simulink model "chris_4R_all_primitives"  (R2024b)
settings: Solver=FixedStepDiscrete  StartTime=0.0  StopTime=60  FixedStep=0.1  MaxStep=0.1  RelTol=1e-3
libraries: neural x220, simulink x1, realtime_pacer_lib x1
(part 8 of 9)

== system chris_4R_all_primitives/RGB to HSV to vel - all robots4/Hue Neural Network/Layer 3/Delays 1 ==
  "p{3}" : Inport  PortDimensions=7
      mask Display: e = 0.06;c1 = [120 230 180]/255;c2 = ([120 230 180]+0)/(256+128);c3 = ([120 230 180]+128)/(256+128);patch([0 1 1 0],[0 0 1 1],c1);patch([0 1 1 1-e 1-e 0+e],[0 0 1 1-e 0+e 0+e],c2);patch([0 0 1 1-e 0+e 0+e],[0 1 1 1-e 1-e 0+e],c3);plot([0 1 1 0 0],[0 0 1 1 0]);
  mux : Mux  Inputs=1
      mask Display: e = 0.06;c1 = [120 150 230]/255;c2 = ([120 150 230]+0)/383;c3 = ([120 150 230]+128)/383;patch([0 1 1 0],[0 0 1 1],c1);patch([0 1 1 1-e 1-e 0+e],[0 0 1 1-e 0+e 0+e],c2);patch([0 0 1 1-e 0+e 0+e],[0 1 1 1-e 1-e 0+e],c3);plot([0 1 1 0 0],[0 0 1 1 0]);disp('Mux')
  "pd{3,2}" : Outport
      mask Display: e = 0.06;c1 = [120 230 180]/255;c2 = ([120 230 180]+0)/(256+128);c3 = ([120 230 180]+128)/(256+128);patch([0 1 1 0],[0 0 1 1],c1);patch([0 1 1 1-e 1-e 0+e],[0 0 1 1-e 0+e 0+e],c2);patch([0 0 1 1-e 0+e 0+e],[0 1 1 1-e 1-e 0+e],c3);plot([0 1 1 0 0],[0 0 1 1 0]);
  wires:
  "p{3}"/1 -> mux/1
  mux/1 -> "pd{3,2}"/1

== system chris_4R_all_primitives/RGB to HSV to vel - all robots4/Hue Neural Network/Layer 3/LW{3,2} ==
  "ad{3,2}" : Inport  PortDimensions=7
      mask Display: e = 0.06;c1 = [120 230 180]/255;c2 = ([120 230 180]+0)/(256+128);c3 = ([120 230 180]+128)/(256+128);patch([0 1 1 0],[0 0 1 1],c1);patch([0 1 1 1-e 1-e 0+e],[0 0 1 1-e 0+e 0+e],c2);patch([0 0 1 1-e 0+e 0+e],[0 1 1 1-e 1-e 0+e],c3);plot([0 1 1 0 0],[0 0 1 1 0]);
  "IW{3,2}(1,:)'" : Constant  Value=[0.2692392715730551611130749734002165496349334716796875;0.176447254974731071452964670243090949952602386474609375;-0.2006583795199970710054770961505710147321224212646484375;0.116348530779392056455634474332327954471111297607421875;0.052531073636257800962834352276331628672778606414794921875;0.02289851615612122082143997658931766636669635772705078125;0.55928841319732980341683514780015684664249420166015625]
      mask Display: e = 0.06;c1 = [120 150 230]/255;c2 = ([120 150 230]+0)/383;c3 = ([120 150 230]+128)/383;patch([0 1 1 0],[0 0 1 1],c1);patch([0 1 1 1-e 1-e 0+e],[0 0 1 1-e 0+e 0+e],c2);patch([0 0 1 1-e 0+e 0+e],[0 1 1 1-e 1-e 0+e],c3);plot([0 1 1 0 0],[0 0 1 1 0]);disp('weights');
  "IW{3,2}(2,:)'" : Constant  Value=[0.2331519658198511202318314872172777540981769561767578125;-0.06009291383108665562939876281234319321811199188232421875;0.440376448501252071299205681498278863728046417236328125;-0.0075677260182224516393834079508451395668089389801025390625;0.3030442642604487257784739995258860290050506591796875;-0.2185483415876194601690230001622694544494152069091796875;0.11610241287844720592392633307099458761513233184814453125]
      mask Display: e = 0.06;c1 = [120 150 230]/255;c2 = ([120 150 230]+0)/383;c3 = ([120 150 230]+128)/383;patch([0 1 1 0],[0 0 1 1],c1);patch([0 1 1 1-e 1-e 0+e],[0 0 1 1-e 0+e 0+e],c2);patch([0 0 1 1-e 0+e 0+e],[0 1 1 1-e 1-e 0+e],c3);plot([0 1 1 0 0],[0 0 1 1 0]);disp('weights');
  Mux : Mux  Inputs=2
      mask Display: e = 0.06;c1 = [120 150 230]/255;c2 = ([120 150 230]+0)/383;c3 = ([120 150 230]+128)/383;patch([0 1 1 0],[0 0 1 1],c1);patch([0 1 1 1-e 1-e 0+e],[0 0 1 1-e 0+e 0+e],c2);patch([0 0 1 1-e 0+e 0+e],[0 1 1 1-e 1-e 0+e],c3);plot([0 1 1 0 0],[0 0 1 1 0]);disp('Mux');
  dotprod1 : neural/Weight Functions/dotprod
  dotprod2 : neural/Weight Functions/dotprod
  "lz{3,2}" : Outport
      mask Display: e = 0.06;c1 = [120 230 180]/255;c2 = ([120 230 180]+0)/(256+128);c3 = ([120 230 180]+128)/(256+128);patch([0 1 1 0],[0 0 1 1],c1);patch([0 1 1 1-e 1-e 0+e],[0 0 1 1-e 0+e 0+e],c2);patch([0 0 1 1-e 0+e 0+e],[0 1 1 1-e 1-e 0+e],c3);plot([0 1 1 0 0],[0 0 1 1 0]);
  wires:
  "IW{3,2}(1,:)'"/1 -> dotprod1/1
  "ad{3,2}"/1 -> dotprod1/2, dotprod2/2
  dotprod1/1 -> Mux/1
  "IW{3,2}(2,:)'"/1 -> dotprod2/1
  dotprod2/1 -> Mux/2
  Mux/1 -> "lz{3,2}"/1

== system chris_4R_all_primitives/RGB to HSV to vel - all robots4/Sat Neural Network/Layer 1/Delays 1 ==
  "p{1}" : Inport  PortDimensions=4
      mask Display: e = 0.06;c1 = [120 230 180]/255;c2 = ([120 230 180]+0)/(256+128);c3 = ([120 230 180]+128)/(256+128);patch([0 1 1 0],[0 0 1 1],c1);patch([0 1 1 1-e 1-e 0+e],[0 0 1 1-e 0+e 0+e],c2);patch([0 0 1 1-e 0+e 0+e],[0 1 1 1-e 1-e 0+e],c3);plot([0 1 1 0 0],[0 0 1 1 0]);
  mux : Mux  Inputs=1
      mask Display: e = 0.06;c1 = [120 150 230]/255;c2 = ([120 150 230]+0)/383;c3 = ([120 150 230]+128)/383;patch([0 1 1 0],[0 0 1 1],c1);patch([0 1 1 1-e 1-e 0+e],[0 0 1 1-e 0+e 0+e],c2);patch([0 0 1 1-e 0+e 0+e],[0 1 1 1-e 1-e 0+e],c3);plot([0 1 1 0 0],[0 0 1 1 0]);disp('Mux')
  "pd{1,1}" : Outport
      mask Display: e = 0.06;c1 = [120 230 180]/255;c2 = ([120 230 180]+0)/(256+128);c3 = ([120 230 180]+128)/(256+128);patch([0 1 1 0],[0 0 1 1],c1);patch([0 1 1 1-e 1-e 0+e],[0 0 1 1-e 0+e 0+e],c2);patch([0 0 1 1-e 0+e 0+e],[0 1 1 1-e 1-e 0+e],c3);plot([0 1 1 0 0],[0 0 1 1 0]);
  wires:
  "p{1}"/1 -> mux/1
  mux/1 -> "pd{1,1}"/1

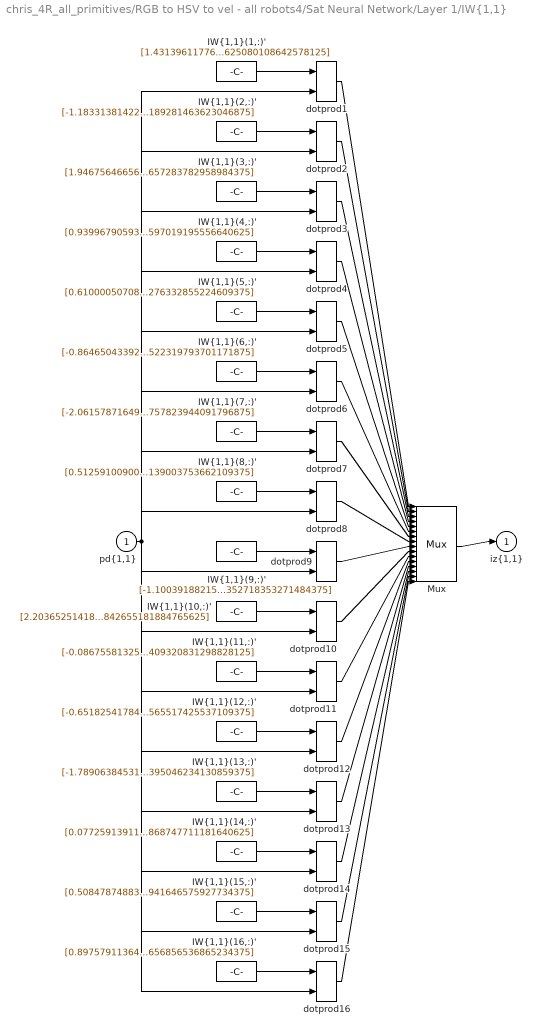
== system chris_4R_all_primitives/RGB to HSV to vel - all robots4/Sat Neural Network/Layer 1/IW{1,1} ==
  "pd{1,1}" : Inport  PortDimensions=4
      mask Display: e = 0.06;c1 = [120 230 180]/255;c2 = ([120 230 180]+0)/(256+128);c3 = ([120 230 180]+128)/(256+128);patch([0 1 1 0],[0 0 1 1],c1);patch([0 1 1 1-e 1-e 0+e],[0 0 1 1-e 0+e 0+e],c2);patch([0 0 1 1-e 0+e 0+e],[0 1 1 1-e 1-e 0+e],c3);plot([0 1 1 0 0],[0 0 1 1 0]);
  "IW{1,1}(1,:)'" : Constant  Value=[1.431396117761938757695361346122808754444122314453125;-2.782058007215437722692286115488968789577484130859375;0.53212897478815468499391272416687570512294769287109375;-1.025242415140987350952173073892481625080108642578125]
      mask Display: e = 0.06;c1 = [120 150 230]/255;c2 = ([120 150 230]+0)/383;c3 = ([120 150 230]+128)/383;patch([0 1 1 0],[0 0 1 1],c1);patch([0 1 1 1-e 1-e 0+e],[0 0 1 1-e 0+e 0+e],c2);patch([0 0 1 1-e 0+e 0+e],[0 1 1 1-e 1-e 0+e],c3);plot([0 1 1 0 0],[0 0 1 1 0]);disp('Weights');
  "IW{1,1}(10,:)'" : Constant  Value=[2.20365251418670649030673303059302270412445068359375;-1.80646533641090822897012913017533719539642333984375;1.0617851828989970375261009394307620823383331298828125;-1.1389975474286606615947903264896012842655181884765625]
      mask Display: e = 0.06;c1 = [120 150 230]/255;c2 = ([120 150 230]+0)/383;c3 = ([120 150 230]+128)/383;patch([0 1 1 0],[0 0 1 1],c1);patch([0 1 1 1-e 1-e 0+e],[0 0 1 1-e 0+e 0+e],c2);patch([0 0 1 1-e 0+e 0+e],[0 1 1 1-e 1-e 0+e],c3);plot([0 1 1 0 0],[0 0 1 1 0]);disp('Weights');
  "IW{1,1}(11,:)'" : Constant  Value=[-0.08675581325626981199494736074484535492956638336181640625;-1.7797064475026489471787272123037837445735931396484375;0.478465586863438707698747975882724858820438385009765625;-2.338810010660509863811284958501346409320831298828125]
      mask Display: e = 0.06;c1 = [120 150 230]/255;c2 = ([120 150 230]+0)/383;c3 = ([120 150 230]+128)/383;patch([0 1 1 0],[0 0 1 1],c1);patch([0 1 1 1-e 1-e 0+e],[0 0 1 1-e 0+e 0+e],c2);patch([0 0 1 1-e 0+e 0+e],[0 1 1 1-e 1-e 0+e],c3);plot([0 1 1 0 0],[0 0 1 1 0]);disp('Weights');
  "IW{1,1}(12,:)'" : Constant  Value=[-0.65182541784813119445374240967794321477413177490234375;0.53703500795189251793004814317100681364536285400390625;1.3713224052105719152905294322408735752105712890625;1.93723084032503489737564450479112565517425537109375]
      mask Display: e = 0.06;c1 = [120 150 230]/255;c2 = ([120 150 230]+0)/383;c3 = ([120 150 230]+128)/383;patch([0 1 1 0],[0 0 1 1],c1);patch([0 1 1 1-e 1-e 0+e],[0 0 1 1-e 0+e 0+e],c2);patch([0 0 1 1-e 0+e 0+e],[0 1 1 1-e 1-e 0+e],c3);plot([0 1 1 0 0],[0 0 1 1 0]);disp('Weights');
  "IW{1,1}(13,:)'" : Constant  Value=[-1.789063845311637646062763451482169330120086669921875;2.29111712274322787408209478599019348621368408203125;0.2900211971528097176786786803859286010265350341796875;-1.6160403812508048471130450707278214395046234130859375]
      mask Display: e = 0.06;c1 = [120 150 230]/255;c2 = ([120 150 230]+0)/383;c3 = ([120 150 230]+128)/383;patch([0 1 1 0],[0 0 1 1],c1);patch([0 1 1 1-e 1-e 0+e],[0 0 1 1-e 0+e 0+e],c2);patch([0 0 1 1-e 0+e 0+e],[0 1 1 1-e 1-e 0+e],c3);plot([0 1 1 0 0],[0 0 1 1 0]);disp('Weights');
  "IW{1,1}(14,:)'" : Constant  Value=[0.07725913911595809480115093492713640443980693817138671875;-1.95190894046138385675703830202110111713409423828125;-1.7302424762236796595971100032329559326171875;-0.86920211937180058558993778206058777868747711181640625]
      mask Display: e = 0.06;c1 = [120 150 230]/255;c2 = ([120 150 230]+0)/383;c3 = ([120 150 230]+128)/383;patch([0 1 1 0],[0 0 1 1],c1);patch([0 1 1 1-e 1-e 0+e],[0 0 1 1-e 0+e 0+e],c2);patch([0 0 1 1-e 0+e 0+e],[0 1 1 1-e 1-e 0+e],c3);plot([0 1 1 0 0],[0 0 1 1 0]);disp('Weights');
  "IW{1,1}(15,:)'" : Constant  Value=[0.50847874883346200203249054538900963962078094482421875;-1.26224358456292673480447774636559188365936279296875;1.7650521246654289342359334114007651805877685546875;0.0124372582914681305277238010376095189712941646575927734375]
      mask Display: e = 0.06;c1 = [120 150 230]/255;c2 = ([120 150 230]+0)/383;c3 = ([120 150 230]+128)/383;patch([0 1 1 0],[0 0 1 1],c1);patch([0 1 1 1-e 1-e 0+e],[0 0 1 1-e 0+e 0+e],c2);patch([0 0 1 1-e 0+e 0+e],[0 1 1 1-e 1-e 0+e],c3);plot([0 1 1 0 0],[0 0 1 1 0]);disp('Weights');
  "IW{1,1}(16,:)'" : Constant  Value=[0.89757911364202536130818543824716471135616302490234375;1.5356735189993122592255758718238212168216705322265625;-1.945340169875237723573491166462190449237823486328125;0.897766214735022938242536838515661656856536865234375]
      mask Display: e = 0.06;c1 = [120 150 230]/255;c2 = ([120 150 230]+0)/383;c3 = ([120 150 230]+128)/383;patch([0 1 1 0],[0 0 1 1],c1);patch([0 1 1 1-e 1-e 0+e],[0 0 1 1-e 0+e 0+e],c2);patch([0 0 1 1-e 0+e 0+e],[0 1 1 1-e 1-e 0+e],c3);plot([0 1 1 0 0],[0 0 1 1 0]);disp('Weights');
  "IW{1,1}(2,:)'" : Constant  Value=[-1.1833138142268133652379447084967978298664093017578125;0.3688515937126377597365944893681444227695465087890625;2.74397295316360345651673924294300377368927001953125;0.413609181588356189518407290961476974189281463623046875]
      mask Display: e = 0.06;c1 = [120 150 230]/255;c2 = ([120 150 230]+0)/383;c3 = ([120 150 230]+128)/383;patch([0 1 1 0],[0 0 1 1],c1);patch([0 1 1 1-e 1-e 0+e],[0 0 1 1-e 0+e 0+e],c2);patch([0 0 1 1-e 0+e 0+e],[0 1 1 1-e 1-e 0+e],c3);plot([0 1 1 0 0],[0 0 1 1 0]);disp('Weights');
  "IW{1,1}(3,:)'" : Constant  Value=[1.9467564665659999878499775149975903332233428955078125;-1.014128041437761140741713461466133594512939453125;-1.1549962182560140622200606230762787163257598876953125;-1.88324456224485370370302916853688657283782958984375]
      mask Display: e = 0.06;c1 = [120 150 230]/255;c2 = ([120 150 230]+0)/383;c3 = ([120 150 230]+128)/383;patch([0 1 1 0],[0 0 1 1],c1);patch([0 1 1 1-e 1-e 0+e],[0 0 1 1-e 0+e 0+e],c2);patch([0 0 1 1-e 0+e 0+e],[0 1 1 1-e 1-e 0+e],c3);plot([0 1 1 0 0],[0 0 1 1 0]);disp('Weights');
  "IW{1,1}(4,:)'" : Constant  Value=[0.93996790593398760194077112828381359577178955078125;-1.15148235769969797814837875193916261196136474609375;1.772533981731274632664963064598850905895233154296875;1.583161624095370090259393691667355597019195556640625]
      mask Display: e = 0.06;c1 = [120 150 230]/255;c2 = ([120 150 230]+0)/383;c3 = ([120 150 230]+128)/383;patch([0 1 1 0],[0 0 1 1],c1);patch([0 1 1 1-e 1-e 0+e],[0 0 1 1-e 0+e 0+e],c2);patch([0 0 1 1-e 0+e 0+e],[0 1 1 1-e 1-e 0+e],c3);plot([0 1 1 0 0],[0 0 1 1 0]);disp('Weights');
  "IW{1,1}(5,:)'" : Constant  Value=[0.6100005070815173180420742937712930142879486083984375;0.7830056954239730249156536956434138119220733642578125;-2.3330503248704150820458380621857941150665283203125;0.9261433624713537593464707242674194276332855224609375]
      mask Display: e = 0.06;c1 = [120 150 230]/255;c2 = ([120 150 230]+0)/383;c3 = ([120 150 230]+128)/383;patch([0 1 1 0],[0 0 1 1],c1);patch([0 1 1 1-e 1-e 0+e],[0 0 1 1-e 0+e 0+e],c2);patch([0 0 1 1-e 0+e 0+e],[0 1 1 1-e 1-e 0+e],c3);plot([0 1 1 0 0],[0 0 1 1 0]);disp('Weights');
  "IW{1,1}(6,:)'" : Constant  Value=[-0.86465043392920615250574201127164997160434722900390625;0.514333377251983581146532742423005402088165283203125;-1.5382261027936348085631834692321717739105224609375;-1.3182065504105491271502614836208522319793701171875]
      mask Display: e = 0.06;c1 = [120 150 230]/255;c2 = ([120 150 230]+0)/383;c3 = ([120 150 230]+128)/383;patch([0 1 1 0],[0 0 1 1],c1);patch([0 1 1 1-e 1-e 0+e],[0 0 1 1-e 0+e 0+e],c2);patch([0 0 1 1-e 0+e 0+e],[0 1 1 1-e 1-e 0+e],c3);plot([0 1 1 0 0],[0 0 1 1 0]);disp('Weights');
  "IW{1,1}(7,:)'" : Constant  Value=[-2.06157871649682444825657512410543859004974365234375;2.342135405773051903821624364354647696018218994140625;0.88344270386245771220501410425640642642974853515625;-1.5034543311927552888818127030390314757823944091796875]
      mask Display: e = 0.06;c1 = [120 150 230]/255;c2 = ([120 150 230]+0)/383;c3 = ([120 150 230]+128)/383;patch([0 1 1 0],[0 0 1 1],c1);patch([0 1 1 1-e 1-e 0+e],[0 0 1 1-e 0+e 0+e],c2);patch([0 0 1 1-e 0+e 0+e],[0 1 1 1-e 1-e 0+e],c3);plot([0 1 1 0 0],[0 0 1 1 0]);disp('Weights');
  "IW{1,1}(8,:)'" : Constant  Value=[0.5125910090030132426619502439280040562152862548828125;1.314277460581450451826412972877733409404754638671875;1.7625328274228733160811088964692316949367523193359375;-1.094697948125618491843624724424444139003753662109375]
      mask Display: e = 0.06;c1 = [120 150 230]/255;c2 = ([120 150 230]+0)/383;c3 = ([120 150 230]+128)/383;patch([0 1 1 0],[0 0 1 1],c1);patch([0 1 1 1-e 1-e 0+e],[0 0 1 1-e 0+e 0+e],c2);patch([0 0 1 1-e 0+e 0+e],[0 1 1 1-e 1-e 0+e],c3);plot([0 1 1 0 0],[0 0 1 1 0]);disp('Weights');
  "IW{1,1}(9,:)'" : Constant  Value=[-1.10039188215190364417139790020883083343505859375;-2.2325332522851457639490035944618284702301025390625;1.278080647177219919541357739944942295551300048828125;0.1841945830369541015070211642523645423352718353271484375]
      mask Display: e = 0.06;c1 = [120 150 230]/255;c2 = ([120 150 230]+0)/383;c3 = ([120 150 230]+128)/383;patch([0 1 1 0],[0 0 1 1],c1);patch([0 1 1 1-e 1-e 0+e],[0 0 1 1-e 0+e 0+e],c2);patch([0 0 1 1-e 0+e 0+e],[0 1 1 1-e 1-e 0+e],c3);plot([0 1 1 0 0],[0 0 1 1 0]);disp('Weights');
  Mux : Mux  Inputs=16
      mask Display: e = 0.06;c1 = [120 150 230]/255;c2 = ([120 150 230]+0)/383;c3 = ([120 150 230]+128)/383;patch([0 1 1 0],[0 0 1 1],c1);patch([0 1 1 1-e 1-e 0+e],[0 0 1 1-e 0+e 0+e],c2);patch([0 0 1 1-e 0+e 0+e],[0 1 1 1-e 1-e 0+e],c3);plot([0 1 1 0 0],[0 0 1 1 0]);disp('Mux');
  dotprod{1..16} (16 alike) : neural/Weight Functions/dotprod
  "iz{1,1}" : Outport
      mask Display: e = 0.06;c1 = [120 230 180]/255;c2 = ([120 230 180]+0)/(256+128);c3 = ([120 230 180]+128)/(256+128);patch([0 1 1 0],[0 0 1 1],c1);patch([0 1 1 1-e 1-e 0+e],[0 0 1 1-e 0+e 0+e],c2);patch([0 0 1 1-e 0+e 0+e],[0 1 1 1-e 1-e 0+e],c3);plot([0 1 1 0 0],[0 0 1 1 0]);
  wires:
  "IW{1,1}(1,:)'"/1 -> dotprod1/1
  "pd{1,1}"/1 -> dotprod1/2, dotprod2/2, dotprod3/2, dotprod4/2, dotprod5/2, dotprod6/2, dotprod7/2, dotprod8/2, dotprod9/2, dotprod10/2, dotprod11/2, dotprod12/2, dotprod13/2, dotprod14/2, dotprod15/2, dotprod16/2
  dotprod1/1 -> Mux/1
  "IW{1,1}(2,:)'"/1 -> dotprod2/1
  dotprod2/1 -> Mux/2
  "IW{1,1}(3,:)'"/1 -> dotprod3/1
  dotprod3/1 -> Mux/3
  "IW{1,1}(4,:)'"/1 -> dotprod4/1
  dotprod4/1 -> Mux/4
  "IW{1,1}(5,:)'"/1 -> dotprod5/1
  dotprod5/1 -> Mux/5
  "IW{1,1}(6,:)'"/1 -> dotprod6/1
  dotprod6/1 -> Mux/6
  "IW{1,1}(7,:)'"/1 -> dotprod7/1
  dotprod7/1 -> Mux/7
  "IW{1,1}(8,:)'"/1 -> dotprod8/1
  dotprod8/1 -> Mux/8
  "IW{1,1}(9,:)'"/1 -> dotprod9/1
  dotprod9/1 -> Mux/9
  "IW{1,1}(10,:)'"/1 -> dotprod10/1
  dotprod10/1 -> Mux/10
  "IW{1,1}(11,:)'"/1 -> dotprod11/1
  dotprod11/1 -> Mux/11
  "IW{1,1}(12,:)'"/1 -> dotprod12/1
  dotprod12/1 -> Mux/12
  "IW{1,1}(13,:)'"/1 -> dotprod13/1
  dotprod13/1 -> Mux/13
  "IW{1,1}(14,:)'"/1 -> dotprod14/1
  dotprod14/1 -> Mux/14
  "IW{1,1}(15,:)'"/1 -> dotprod15/1
  dotprod15/1 -> Mux/15
  "IW{1,1}(16,:)'"/1 -> dotprod16/1
  dotprod16/1 -> Mux/16
  Mux/1 -> "iz{1,1}"/1

== system chris_4R_all_primitives/RGB to HSV to vel - all robots4/Sat Neural Network/Layer 2/Delays 1 ==
  "p{2}" : Inport  PortDimensions=16
      mask Display: e = 0.06;c1 = [120 230 180]/255;c2 = ([120 230 180]+0)/(256+128);c3 = ([120 230 180]+128)/(256+128);patch([0 1 1 0],[0 0 1 1],c1);patch([0 1 1 1-e 1-e 0+e],[0 0 1 1-e 0+e 0+e],c2);patch([0 0 1 1-e 0+e 0+e],[0 1 1 1-e 1-e 0+e],c3);plot([0 1 1 0 0],[0 0 1 1 0]);
  mux : Mux  Inputs=1
      mask Display: e = 0.06;c1 = [120 150 230]/255;c2 = ([120 150 230]+0)/383;c3 = ([120 150 230]+128)/383;patch([0 1 1 0],[0 0 1 1],c1);patch([0 1 1 1-e 1-e 0+e],[0 0 1 1-e 0+e 0+e],c2);patch([0 0 1 1-e 0+e 0+e],[0 1 1 1-e 1-e 0+e],c3);plot([0 1 1 0 0],[0 0 1 1 0]);disp('Mux')
  "pd{2,1}" : Outport
      mask Display: e = 0.06;c1 = [120 230 180]/255;c2 = ([120 230 180]+0)/(256+128);c3 = ([120 230 180]+128)/(256+128);patch([0 1 1 0],[0 0 1 1],c1);patch([0 1 1 1-e 1-e 0+e],[0 0 1 1-e 0+e 0+e],c2);patch([0 0 1 1-e 0+e 0+e],[0 1 1 1-e 1-e 0+e],c3);plot([0 1 1 0 0],[0 0 1 1 0]);
  wires:
  "p{2}"/1 -> mux/1
  mux/1 -> "pd{2,1}"/1

== system chris_4R_all_primitives/RGB to HSV to vel - all robots4/Sat Neural Network/Layer 2/LW{2,1} ==
  "ad{2,1}" : Inport  PortDimensions=16
      mask Display: e = 0.06;c1 = [120 230 180]/255;c2 = ([120 230 180]+0)/(256+128);c3 = ([120 230 180]+128)/(256+128);patch([0 1 1 0],[0 0 1 1],c1);patch([0 1 1 1-e 1-e 0+e],[0 0 1 1-e 0+e 0+e],c2);patch([0 0 1 1-e 0+e 0+e],[0 1 1 1-e 1-e 0+e],c3);plot([0 1 1 0 0],[0 0 1 1 0]);
  "IW{2,1}(1,:)'" : Constant  Value=[0.0405182376918509501440013309547794051468372344970703125;-0.2005965242417274974062735282132052816450595855712890625;-0.288052399058029318101858962108963169157505035400390625;-0.033798797939179357763261890568173839710652828216552734375;-0.38873917912712740996283855565707199275493621826171875;-0.388040345257807561818452768420684151351451873779296875;0.299933426047902795819055654646945185959339141845703125;-0.1027435018404385669299472283455543220043182373046875;-0.583009164015153569238236741512082517147064208984375;-0.78193931272048045055811371639720164239406585693359375;-0.65708008842550869044174532973556779325008392333984375;0.10191008257822946336812464096510666422545909881591796875;-0.23833579598253196163426537168561480939388275146484375;0.6103221938149105962878593345521949231624603271484375;0.399453160369107440619274029813823290169239044189453125;-0.185472773287069292447171164894825778901576995849609375]
      mask Display: e = 0.06;c1 = [120 150 230]/255;c2 = ([120 150 230]+0)/383;c3 = ([120 150 230]+128)/383;patch([0 1 1 0],[0 0 1 1],c1);patch([0 1 1 1-e 1-e 0+e],[0 0 1 1-e 0+e 0+e],c2);patch([0 0 1 1-e 0+e 0+e],[0 1 1 1-e 1-e 0+e],c3);plot([0 1 1 0 0],[0 0 1 1 0]);disp('weights');
  "IW{2,1}(10,:)'" : Constant  Value=[-0.452191701750555397065767238018452189862728118896484375;-0.0221133050903745027870872519315526005811989307403564453125;-0.50668042109564515040887044960982166230678558349609375;-0.134466263597315005551280364670674316585063934326171875;-0.5778872938558474725567748464527539908885955810546875;-0.330090590163657437994260135383228771388530731201171875;-0.88211729209087208491979481550515629351139068603515625;0.05704723886842806568342467699039843864738941192626953125;-0.457686002713864670266019629707443527877330780029296875;-0.363545538448391436503470686147920787334442138671875;-0.46792752643960888736529568632249720394611358642578125;-0.374745597525016627127314450262929312884807586669921875;0.420307988899386142378489239490590989589691162109375;0.67587757484243715655480855275527574121952056884765625;-0.332056332006116783350790910844807513058185577392578125;0.262509964419624763909411058193654753267765045166015625]
      mask Display: e = 0.06;c1 = [120 150 230]/255;c2 = ([120 150 230]+0)/383;c3 = ([120 150 230]+128)/383;patch([0 1 1 0],[0 0 1 1],c1);patch([0 1 1 1-e 1-e 0+e],[0 0 1 1-e 0+e 0+e],c2);patch([0 0 1 1-e 0+e 0+e],[0 1 1 1-e 1-e 0+e],c3);plot([0 1 1 0 0],[0 0 1 1 0]);disp('weights');
  "IW{2,1}(11,:)'" : Constant  Value=[0.45306980562450049898615134225110523402690887451171875;-0.1337506557395084227923831576845259405672550201416015625;0.5804219089400752817908823999459855258464813232421875;0.6619766068517132229231947349035181105136871337890625;0.51277027566559973958959517403854988515377044677734375;-0.2207933461218836435069334811487351544201374053955078125;0.0859082911000610405238830935559235513210296630859375;-0.099394914399163425411387606800417415797710418701171875;-0.59019989641980019623446196419536136090755462646484375;-0.328545597534417532781247928141965530812740325927734375;0.45857226435172149248131745480350218713283538818359375;0.82963816647782950841616411707946099340915679931640625;0.76267013234799918564021936617791652679443359375;0.2353473942266718632598809790579252876341342926025390625;-0.3234191811884838951840492882183752954006195068359375;0.23807432623823554518338596608373336493968963623046875]
      mask Display: e = 0.06;c1 = [120 150 230]/255;c2 = ([120 150 230]+0)/383;c3 = ([120 150 230]+128)/383;patch([0 1 1 0],[0 0 1 1],c1);patch([0 1 1 1-e 1-e 0+e],[0 0 1 1-e 0+e 0+e],c2);patch([0 0 1 1-e 0+e 0+e],[0 1 1 1-e 1-e 0+e],c3);plot([0 1 1 0 0],[0 0 1 1 0]);disp('weights');
  "IW{2,1}(2,:)'" : Constant  Value=[0.288539306225060465660448016933514736592769622802734375;-0.51576248108568611971946893390850163996219635009765625;0.45424885669401737775530136786983348429203033447265625;0.5298492013146456347527646357775665819644927978515625;-0.1819345119646678110569837372167967259883880615234375;-0.285600495543814225651857441334868781268596649169921875;0.464339645797900046897410675228456966578960418701171875;-0.58206428193664228043502362197614274919033050537109375;0.51913641430267143395127504845731891691684722900390625;-0.235906014205401304284492880469770170748233795166015625;-0.446102812988154850959432451418251730501651763916015625;0.43556849597498814574692005407996475696563720703125;-0.177910205398422005540481904972693882882595062255859375;0.54608901806667964340391563382581807672977447509765625;-0.10922386742774008172585098463969188742339611053466796875;-0.040425042947252957936665751503824139945209026336669921875]
      mask Display: e = 0.06;c1 = [120 150 230]/255;c2 = ([120 150 230]+0)/383;c3 = ([120 150 230]+128)/383;patch([0 1 1 0],[0 0 1 1],c1);patch([0 1 1 1-e 1-e 0+e],[0 0 1 1-e 0+e 0+e],c2);patch([0 0 1 1-e 0+e 0+e],[0 1 1 1-e 1-e 0+e],c3);plot([0 1 1 0 0],[0 0 1 1 0]);disp('weights');
  "IW{2,1}(3,:)'" : Constant  Value=[-0.36786108382063187338673060367000289261341094970703125;-0.005099256166760724080788680367959386785514652729034423828125;0.61749781127701197647184017114341259002685546875;0.07853379202744663334367913876121747307479381561279296875;0.02886539838621733633505783700456959195435047149658203125;-0.08146341803118177515852238457227940671145915985107421875;-0.33731387144394109345313381709274835884571075439453125;-0.6259262003198664547909402244840748608112335205078125;0.08636088100819873381031044345945701934397220611572265625;0.26005482094589649211258119976264424622058868408203125;0.1517762222498661717207113497352111153304576873779296875;-0.45921912494541283766835704227560199797153472900390625;0.81073080042589562577148853961261920630931854248046875;-0.162105728366866319589689737767912447452545166015625;0.327104347832572195375888668422703631222248077392578125;0.240254515359306253241555850763688795268535614013671875]
      mask Display: e = 0.06;c1 = [120 150 230]/255;c2 = ([120 150 230]+0)/383;c3 = ([120 150 230]+128)/383;patch([0 1 1 0],[0 0 1 1],c1);patch([0 1 1 1-e 1-e 0+e],[0 0 1 1-e 0+e 0+e],c2);patch([0 0 1 1-e 0+e 0+e],[0 1 1 1-e 1-e 0+e],c3);plot([0 1 1 0 0],[0 0 1 1 0]);disp('weights');
  "IW{2,1}(4,:)'" : Constant  Value=[-0.87068543923802554918012219786760397255420684814453125;-0.836564203865024058615063040633685886859893798828125;-0.310062225313615102972875092746107839047908782958984375;-0.06989088281138820801796640580505481921136379241943359375;1.21004359065693289920773167978040874004364013671875;0.81780629717440478376744295019307173788547515869140625;1.0113275013996541051852773307473398745059967041015625;-0.2143563929170544113400609376185457222163677215576171875;-0.73571406072879519388862945561413653194904327392578125;0.95303194700619064949620451443479396402835845947265625;-0.54623655564589557176446987796225585043430328369140625;0.26990522703693908823652236605994403362274169921875;-0.7026265580688895173722130493842996656894683837890625;0.1739410748171972276310270899557508528232574462890625;-0.42446015924387181517118960982770659029483795166015625;0.41739860008352913656182181512122042477130889892578125]
      mask Display: e = 0.06;c1 = [120 150 230]/255;c2 = ([120 150 230]+0)/383;c3 = ([120 150 230]+128)/383;patch([0 1 1 0],[0 0 1 1],c1);patch([0 1 1 1-e 1-e 0+e],[0 0 1 1-e 0+e 0+e],c2);patch([0 0 1 1-e 0+e 0+e],[0 1 1 1-e 1-e 0+e],c3);plot([0 1 1 0 0],[0 0 1 1 0]);disp('weights');
  "IW{2,1}(5,:)'" : Constant  Value=[0.2118177713413592344604552408782183192670345306396484375;0.0440596735797484650998256938692065887153148651123046875;0.1504709240944588077848464990893262438476085662841796875;0.1154582573993709060378165531801641918718814849853515625;0.372976931374041142941422322110156528651714324951171875;0.18907196399340497894314694349304772913455963134765625;-0.71772819162937351311626343886018730700016021728515625;0.29824366855064698977884063424426130950450897216796875;0.5477614405142718911889687660732306540012359619140625;-0.430119329693274654591306216389057226479053497314453125;-0.38898311876392754893316805464564822614192962646484375;-0.295146535133338605572106416730093769729137420654296875;-0.59218974603233609510510859763599000871181488037109375;0.223108009443776900138090013570035807788372039794921875;-0.5946835093901092772483707449282519519329071044921875;0.53233051422360289084423357053310610353946685791015625]
      mask Display: e = 0.06;c1 = [120 150 230]/255;c2 = ([120 150 230]+0)/383;c3 = ([120 150 230]+128)/383;patch([0 1 1 0],[0 0 1 1],c1);patch([0 1 1 1-e 1-e 0+e],[0 0 1 1-e 0+e 0+e],c2);patch([0 0 1 1-e 0+e 0+e],[0 1 1 1-e 1-e 0+e],c3);plot([0 1 1 0 0],[0 0 1 1 0]);disp('weights');
  "IW{2,1}(6,:)'" : Constant  Value=[-0.3914118560140185110185484518297016620635986328125;0.16870621398827234660444673863821662962436676025390625;-0.62539033872283333881370026574586518108844757080078125;0.2016700473586527653235833668077248148620128631591796875;-0.53790130235048660978236512164585292339324951171875;0.0048816685664508606412592683909679180942475795745849609375;0.69648905086128654051691455606487579643726348876953125;-0.424951234840228619926705277975997887551784515380859375;-0.31327775134513247135004121446399949491024017333984375;0.7395220884008579798063465204904787242412567138671875;-0.8247851923713067634480466949753463268280029296875;-0.05268243132451806698401952644417178817093372344970703125;-0.23524491584177320557813573032035492360591888427734375;-0.69704527818500483515862242711591534316539764404296875;-0.409597217410627878475537499980418942868709564208984375;0.5218245929004636796122440500766970217227935791015625]
      mask Display: e = 0.06;c1 = [120 150 230]/255;c2 = ([120 150 230]+0)/383;c3 = ([120 150 230]+128)/383;patch([0 1 1 0],[0 0 1 1],c1);patch([0 1 1 1-e 1-e 0+e],[0 0 1 1-e 0+e 0+e],c2);patch([0 0 1 1-e 0+e 0+e],[0 1 1 1-e 1-e 0+e],c3);plot([0 1 1 0 0],[0 0 1 1 0]);disp('weights');
  "IW{2,1}(7,:)'" : Constant  Value=[-0.31461581947257888369762213187641464173793792724609375;0.8640159316636604192041204441920854151248931884765625;-0.468804948094664053481750443097553215920925140380859375;0.38414201749038190403240378145710565149784088134765625;-0.92076324232259942892397930336301214993000030517578125;0.13541754487057555689233367957058362662792205810546875;-0.450716375509893352191426174613297916948795318603515625;-0.34999345932768421985059603684931062161922454833984375;0.51033294463980405364367243237211368978023529052734375;0.1694379412702841924964758391070063225924968719482421875;0.40710095474024832196136003403807990252971649169921875;0.07852206101797708226452954249907634221017360687255859375;0.326875798371287606958190963268862105906009674072265625;-0.185007392601754416805448499871999956667423248291015625;-0.33567542425687679763512960562366060912609100341796875;0.12068755201098746443477693901513703167438507080078125]
      mask Display: e = 0.06;c1 = [120 150 230]/255;c2 = ([120 150 230]+0)/383;c3 = ([120 150 230]+128)/383;patch([0 1 1 0],[0 0 1 1],c1);patch([0 1 1 1-e 1-e 0+e],[0 0 1 1-e 0+e 0+e],c2);patch([0 0 1 1-e 0+e 0+e],[0 1 1 1-e 1-e 0+e],c3);plot([0 1 1 0 0],[0 0 1 1 0]);disp('weights');
  "IW{2,1}(8,:)'" : Constant  Value=[0.1590453079257107826816053375296178273856639862060546875;1.0459805433733018187325569670065306127071380615234375;0.215600065266059404134324495316832326352596282958984375;-0.410652046602745457448691013269126415252685546875;-0.78449977288274597153616696232347749173641204833984375;0.2352102495180614372127791966704535298049449920654296875;-1.739785799559422141413733697845600545406341552734375;0.05716354815408364320461487295688129961490631103515625;0.24692707662855373218491195075330324470996856689453125;-0.08690243856649504383682369734742678701877593994140625;-0.118235408064418956453067721668048761785030364990234375;0.0263063700406527441189030724899566848762333393096923828125;-0.23623100233663674174522384419105947017669677734375;-0.0651182255830201894841735565933049656450748443603515625;0.214300864470770624503614953937358222901821136474609375;-0.75694612009589901102657449882826767861843109130859375]
      mask Display: e = 0.06;c1 = [120 150 230]/255;c2 = ([120 150 230]+0)/383;c3 = ([120 150 230]+128)/383;patch([0 1 1 0],[0 0 1 1],c1);patch([0 1 1 1-e 1-e 0+e],[0 0 1 1-e 0+e 0+e],c2);patch([0 0 1 1-e 0+e 0+e],[0 1 1 1-e 1-e 0+e],c3);plot([0 1 1 0 0],[0 0 1 1 0]);disp('weights');
  "IW{2,1}(9,:)'" : Constant  Value=[-0.545527523742709963272545792278833687305450439453125;0.5766714855953958274170645381673239171504974365234375;-0.76528559402613882678423351535457186400890350341796875;0.09830036236684935868623824717360548675060272216796875;-0.08070535020050968733063001536720548756420612335205078125;-0.08798823799328425732113601043238304555416107177734375;0.424530264888417774304940621732384897768497467041015625;-0.3847717864829858225306224994710646569728851318359375;-0.256571594989565665567710084360442124307155609130859375;-0.5461473812368555780238921215641312301158905029296875;0.5944160275387158076654259275528602302074432373046875;-0.072939095747945603687156790329026989638805389404296875;0.7688499294743451617506480033625848591327667236328125;0.210655594234719745205808294485905207693576812744140625;-0.469219178452916441113274004237609915435314178466796875;-0.8445603243351766931112933889380656182765960693359375]
      mask Display: e = 0.06;c1 = [120 150 230]/255;c2 = ([120 150 230]+0)/383;c3 = ([120 150 230]+128)/383;patch([0 1 1 0],[0 0 1 1],c1);patch([0 1 1 1-e 1-e 0+e],[0 0 1 1-e 0+e 0+e],c2);patch([0 0 1 1-e 0+e 0+e],[0 1 1 1-e 1-e 0+e],c3);plot([0 1 1 0 0],[0 0 1 1 0]);disp('weights');
  Mux : Mux  Inputs=11
      mask Display: e = 0.06;c1 = [120 150 230]/255;c2 = ([120 150 230]+0)/383;c3 = ([120 150 230]+128)/383;patch([0 1 1 0],[0 0 1 1],c1);patch([0 1 1 1-e 1-e 0+e],[0 0 1 1-e 0+e 0+e],c2);patch([0 0 1 1-e 0+e 0+e],[0 1 1 1-e 1-e 0+e],c3);plot([0 1 1 0 0],[0 0 1 1 0]);disp('Mux');
  dotprod{1..11} (11 alike) : neural/Weight Functions/dotprod
  "lz{2,1}" : Outport
      mask Display: e = 0.06;c1 = [120 230 180]/255;c2 = ([120 230 180]+0)/(256+128);c3 = ([120 230 180]+128)/(256+128);patch([0 1 1 0],[0 0 1 1],c1);patch([0 1 1 1-e 1-e 0+e],[0 0 1 1-e 0+e 0+e],c2);patch([0 0 1 1-e 0+e 0+e],[0 1 1 1-e 1-e 0+e],c3);plot([0 1 1 0 0],[0 0 1 1 0]);
  wires:
  "IW{2,1}(1,:)'"/1 -> dotprod1/1
  "ad{2,1}"/1 -> dotprod1/2, dotprod2/2, dotprod3/2, dotprod4/2, dotprod5/2, dotprod6/2, dotprod7/2, dotprod8/2, dotprod9/2, dotprod10/2, dotprod11/2
  dotprod1/1 -> Mux/1
  "IW{2,1}(2,:)'"/1 -> dotprod2/1
  dotprod2/1 -> Mux/2
  "IW{2,1}(3,:)'"/1 -> dotprod3/1
  dotprod3/1 -> Mux/3
  "IW{2,1}(4,:)'"/1 -> dotprod4/1
  dotprod4/1 -> Mux/4
  "IW{2,1}(5,:)'"/1 -> dotprod5/1
  dotprod5/1 -> Mux/5
  "IW{2,1}(6,:)'"/1 -> dotprod6/1
  dotprod6/1 -> Mux/6
  "IW{2,1}(7,:)'"/1 -> dotprod7/1
  dotprod7/1 -> Mux/7
  "IW{2,1}(8,:)'"/1 -> dotprod8/1
  dotprod8/1 -> Mux/8
  "IW{2,1}(9,:)'"/1 -> dotprod9/1
  dotprod9/1 -> Mux/9
  "IW{2,1}(10,:)'"/1 -> dotprod10/1
  dotprod10/1 -> Mux/10
  "IW{2,1}(11,:)'"/1 -> dotprod11/1
  dotprod11/1 -> Mux/11
  Mux/1 -> "lz{2,1}"/1

== system chris_4R_all_primitives/RGB to HSV to vel - all robots4/Sat Neural Network/Layer 3/Delays 1 ==
  "p{3}" : Inport  PortDimensions=11
      mask Display: e = 0.06;c1 = [120 230 180]/255;c2 = ([120 230 180]+0)/(256+128);c3 = ([120 230 180]+128)/(256+128);patch([0 1 1 0],[0 0 1 1],c1);patch([0 1 1 1-e 1-e 0+e],[0 0 1 1-e 0+e 0+e],c2);patch([0 0 1 1-e 0+e 0+e],[0 1 1 1-e 1-e 0+e],c3);plot([0 1 1 0 0],[0 0 1 1 0]);
  mux : Mux  Inputs=1
      mask Display: e = 0.06;c1 = [120 150 230]/255;c2 = ([120 150 230]+0)/383;c3 = ([120 150 230]+128)/383;patch([0 1 1 0],[0 0 1 1],c1);patch([0 1 1 1-e 1-e 0+e],[0 0 1 1-e 0+e 0+e],c2);patch([0 0 1 1-e 0+e 0+e],[0 1 1 1-e 1-e 0+e],c3);plot([0 1 1 0 0],[0 0 1 1 0]);disp('Mux')
  "pd{3,2}" : Outport
      mask Display: e = 0.06;c1 = [120 230 180]/255;c2 = ([120 230 180]+0)/(256+128);c3 = ([120 230 180]+128)/(256+128);patch([0 1 1 0],[0 0 1 1],c1);patch([0 1 1 1-e 1-e 0+e],[0 0 1 1-e 0+e 0+e],c2);patch([0 0 1 1-e 0+e 0+e],[0 1 1 1-e 1-e 0+e],c3);plot([0 1 1 0 0],[0 0 1 1 0]);
  wires:
  "p{3}"/1 -> mux/1
  mux/1 -> "pd{3,2}"/1

== system chris_4R_all_primitives/RGB to HSV to vel - all robots4/Sat Neural Network/Layer 3/LW{3,2} ==
  "ad{3,2}" : Inport  PortDimensions=11
      mask Display: e = 0.06;c1 = [120 230 180]/255;c2 = ([120 230 180]+0)/(256+128);c3 = ([120 230 180]+128)/(256+128);patch([0 1 1 0],[0 0 1 1],c1);patch([0 1 1 1-e 1-e 0+e],[0 0 1 1-e 0+e 0+e],c2);patch([0 0 1 1-e 0+e 0+e],[0 1 1 1-e 1-e 0+e],c3);plot([0 1 1 0 0],[0 0 1 1 0]);
  "IW{3,2}(1,:)'" : Constant  Value=[-0.63093613889335331545993312829523347318172454833984375;-0.2981907598877686638161321752704679965972900390625;0.67501205269705000233670943998731672763824462890625;-1.6833932169586300897634600914898328483104705810546875;0.2104658793440022657161847519091679714620113372802734375;-0.4684746928622935957520212468807585537433624267578125;-0.43341066969200381375770803060731850564479827880859375;-0.87971961349906646621121808493626303970813751220703125;0.47369942446536150715274970934842713177204132080078125;0.60240331306595107374590725157759152352809906005859375;0.368481191649497719087236191626288928091526031494140625]
      mask Display: e = 0.06;c1 = [120 150 230]/255;c2 = ([120 150 230]+0)/383;c3 = ([120 150 230]+128)/383;patch([0 1 1 0],[0 0 1 1],c1);patch([0 1 1 1-e 1-e 0+e],[0 0 1 1-e 0+e 0+e],c2);patch([0 0 1 1-e 0+e 0+e],[0 1 1 1-e 1-e 0+e],c3);plot([0 1 1 0 0],[0 0 1 1 0]);disp('weights');
  Mux : Mux  Inputs=1
      mask Display: e = 0.06;c1 = [120 150 230]/255;c2 = ([120 150 230]+0)/383;c3 = ([120 150 230]+128)/383;patch([0 1 1 0],[0 0 1 1],c1);patch([0 1 1 1-e 1-e 0+e],[0 0 1 1-e 0+e 0+e],c2);patch([0 0 1 1-e 0+e 0+e],[0 1 1 1-e 1-e 0+e],c3);plot([0 1 1 0 0],[0 0 1 1 0]);disp('Mux');
  dotprod1 : neural/Weight Functions/dotprod
  "lz{3,2}" : Outport
      mask Display: e = 0.06;c1 = [120 230 180]/255;c2 = ([120 230 180]+0)/(256+128);c3 = ([120 230 180]+128)/(256+128);patch([0 1 1 0],[0 0 1 1],c1);patch([0 1 1 1-e 1-e 0+e],[0 0 1 1-e 0+e 0+e],c2);patch([0 0 1 1-e 0+e 0+e],[0 1 1 1-e 1-e 0+e],c3);plot([0 1 1 0 0],[0 0 1 1 0]);
  wires:
  "IW{3,2}(1,:)'"/1 -> dotprod1/1
  "ad{3,2}"/1 -> dotprod1/2
  dotprod1/1 -> Mux/1
  Mux/1 -> "lz{3,2}"/1

== matlab function chris_4R_all_primitives/Robot_signal_processing_4/Global to Body Rotation Matrix ==
  data: u input; y output
function y = fcn(u)

y = [cos(u) -sin(u) 0; sin(u) cos(u) 0; 0 0 1];

== matlab function chris_4R_all_primitives/RGB to HSV to vel - all robots1/RGB to HSV ==
  data: R output; G output; B output; K output; R input; G input; B input; K input
function [R, G, B, K]= data_augmentation(R, G, B, K)

  R = squeeze(R);
  G = squeeze(G); 
  B = squeeze(B);
  K = squeeze(K);
  
   
  % Normalize RGB to [0, 1]
    R = (R - 120) / 1300;
    G = (G - 120) / 1300;
    B = (B - 120) / 1300;
    K = (K - 800) / 3500;

    R = max(min(R, 1), 0);
    G = max(min(G, 1), 0);
    B = max(min(B, 1), 0);
    K = max(min(K, 1), 0);

    Cmax = max(max(R, G), B);
    Cmin = min(min(R, G), B);
    delta = Cmax - Cmin;

end

== matlab function chris_4R_all_primitives/RGB to HSV to vel - all robots1/hue_post_processor ==
  data: hue output; hue_nn_sin input; hue_nn_cos input
function hue = hue_post_processing(hue_nn_sin, hue_nn_cos)

hue_nn_sin = (hue_nn_sin+1)/2;
hue_nn_cos = (hue_nn_cos+1)/2;

hue = atan2(hue_nn_sin, hue_nn_cos);
hue(hue < 0) = hue(hue < 0) + 2 * pi;
hue = hue / (2 * pi);


hue = max(0,min(hue,1));
end

== matlab function chris_4R_all_primitives/RGB to HSV to vel - all robots1/sat_post_processor ==
  data: sat output; sat_nn_output input
function sat = sat_post_processing(sat_nn_output)

sat = (sat_nn_output+1)/2;

sat = max(0,min(sat,1));
end

== matlab function chris_4R_all_primitives/RGB to HSV to vel - all robots1/sat_post_processor1 ==
  data: data output; data_raw input
function data = data_normalizing(data_raw)

data = (data_raw*2)-1;


end

== matlab function chris_4R_all_primitives/RGB to HSV to vel - all robots2/RGB to HSV ==
  data: R output; G output; B output; K output; R input; G input; B input; K input
function [R, G, B, K]= data_augmentation(R, G, B, K)

  R = squeeze(R);
  G = squeeze(G); 
  B = squeeze(B);
  K = squeeze(K);
  
   
  % Normalize RGB to [0, 1]
    R = (R - 120) / 1300;
    G = (G - 120) / 1300;
    B = (B - 120) / 1300;
    K = (K - 800) / 3500;

    R = max(min(R, 1), 0);
    G = max(min(G, 1), 0);
    B = max(min(B, 1), 0);
    K = max(min(K, 1), 0);

    Cmax = max(max(R, G), B);
    Cmin = min(min(R, G), B);
    delta = Cmax - Cmin;

end

== matlab function chris_4R_all_primitives/RGB to HSV to vel - all robots2/hue_post_processor ==
  data: hue output; hue_nn_sin input; hue_nn_cos input
function hue = hue_post_processing(hue_nn_sin, hue_nn_cos)

hue_nn_sin = (hue_nn_sin+1)/2;
hue_nn_cos = (hue_nn_cos+1)/2;

hue = atan2(hue_nn_sin, hue_nn_cos);
hue(hue < 0) = hue(hue < 0) + 2 * pi;
hue = hue / (2 * pi);


hue = max(0,min(hue,1));
end

== matlab function chris_4R_all_primitives/RGB to HSV to vel - all robots2/sat_post_processor ==
  data: sat output; sat_nn_output input
function sat = sat_post_processing(sat_nn_output)

sat = (sat_nn_output+1)/2;

sat = max(0,min(sat,1));
end

== matlab function chris_4R_all_primitives/RGB to HSV to vel - all robots2/sat_post_processor1 ==
  data: data output; data_raw input
function data = data_normalizing(data_raw)

data = (data_raw*2)-1;


end

== matlab function chris_4R_all_primitives/RGB to HSV to vel - all robots3/RGB to HSV ==
  data: R output; G output; B output; K output; R input; G input; B input; K input
function [R, G, B, K]= data_augmentation(R, G, B, K)

  R = squeeze(R);
  G = squeeze(G); 
  B = squeeze(B);
  K = squeeze(K);
  
   
  % Normalize RGB to [0, 1]
    R = (R - 120) / 1300;
    G = (G - 120) / 1300;
    B = (B - 120) / 1300;
    K = (K - 800) / 3500;

    R = max(min(R, 1), 0);
    G = max(min(G, 1), 0);
    B = max(min(B, 1), 0);
    K = max(min(K, 1), 0);

    Cmax = max(max(R, G), B);
    Cmin = min(min(R, G), B);
    delta = Cmax - Cmin;

end

== matlab function chris_4R_all_primitives/RGB to HSV to vel - all robots3/hue_post_processor ==
  data: hue output; hue_nn_sin input; hue_nn_cos input
function hue = hue_post_processing(hue_nn_sin, hue_nn_cos)

hue_nn_sin = (hue_nn_sin+1)/2;
hue_nn_cos = (hue_nn_cos+1)/2;

hue = atan2(hue_nn_sin, hue_nn_cos);
hue(hue < 0) = hue(hue < 0) + 2 * pi;
hue = hue / (2 * pi);


hue = max(0,min(hue,1));
end

== matlab function chris_4R_all_primitives/RGB to HSV to vel - all robots3/sat_post_processor ==
  data: sat output; sat_nn_output input
function sat = sat_post_processing(sat_nn_output)

sat = (sat_nn_output+1)/2;

sat = max(0,min(sat,1));
end

== matlab function chris_4R_all_primitives/RGB to HSV to vel - all robots3/sat_post_processor1 ==
  data: data output; data_raw input
function data = data_normalizing(data_raw)

data = (data_raw*2)-1;


end

== matlab function chris_4R_all_primitives/RGB to HSV to vel - all robots4/RGB to HSV ==
  data: R output; G output; B output; K output; R input; G input; B input; K input
function [R, G, B, K]= data_augmentation(R, G, B, K)

  R = squeeze(R);
  G = squeeze(G); 
  B = squeeze(B);
  K = squeeze(K);
  
   
  % Normalize RGB to [0, 1]
    R = (R - 120) / 1300;
    G = (G - 120) / 1300;
    B = (B - 120) / 1300;
    K = (K - 800) / 3500;

    R = max(min(R, 1), 0);
    G = max(min(G, 1), 0);
    B = max(min(B, 1), 0);
    K = max(min(K, 1), 0);

    Cmax = max(max(R, G), B);
    Cmin = min(min(R, G), B);
    delta = Cmax - Cmin;

end

== matlab function chris_4R_all_primitives/RGB to HSV to vel - all robots4/hue_post_processor ==
  data: hue output; hue_nn_sin input; hue_nn_cos input
function hue = hue_post_processing(hue_nn_sin, hue_nn_cos)

hue_nn_sin = (hue_nn_sin+1)/2;
hue_nn_cos = (hue_nn_cos+1)/2;

hue = atan2(hue_nn_sin, hue_nn_cos);
hue(hue < 0) = hue(hue < 0) + 2 * pi;
hue = hue / (2 * pi);


hue = max(0,min(hue,1));
end

== matlab function chris_4R_all_primitives/RGB to HSV to vel - all robots4/sat_post_processor ==
  data: sat output; sat_nn_output input
function sat = sat_post_processing(sat_nn_output)

sat = (sat_nn_output+1)/2;

sat = max(0,min(sat,1));
end

== matlab function chris_4R_all_primitives/RGB to HSV to vel - all robots4/sat_post_processor1 ==
  data: data output; data_raw input
function data = data_normalizing(data_raw)

data = (data_raw*2)-1;


end

== matlab function chris_4R_all_primitives/Jacobians/Cartesian to Cluster Variables ==
  data: fwdkin output; x1 input; x_c output; y1 input; th1 input; x2 input; y2 input; th2 input; x3 input; y3 input; th3 input; y_c output; th_c output; d1 output; d2 output; r1 output; x4 input; y4 input; r2 output; phi output; th4 input
function [fwdkin, x_c, y_c, th_c, d1, d2, r1, r2, phi] = Forward_Kinematics(x1, y1, th1, x2, y2, th2, x3, y3, th3, x4, y4, th4)
% Forward_Kinematics: Convert corner coordinates to diagonal parameters
% 
% Inputs:
%   x1, y1, th1: Position and orientation of corner 1
%   x2, y2, th2: Position and orientation of corner 2  
%   x3, y3, th3: Position and orientation of corner 3
%   x4, y4, th4: Position and orientation of corner 4
%
% Outputs:
%   fwdkin: [d1, d2, r1, r2, phi, x_c, y_c, th_c] - diagonal parameters
%   x_c, y_c: Centroid coordinates
%   th_c: Overall rotation angle (theta)
%   d1, d2: Diagonal lengths
%   r1, r2: Intersection ratios
%   theta_1: Same as th_c (for compatibility)

% Centre frame (centroid)
x_c = (x1 + x2 + x3 + x4) / 4;
y_c = (y1 + y2 + y3 + y4) / 4;

% Diagonal lengths
d1 = sqrt((x3 - x1)^2 + (y3 - y1)^2);  % Diagonal 1-3
d2 = sqrt((x4 - x2)^2 + (y4 - y2)^2);  % Diagonal 2-4

%% Swapping this part out
% Overall rotation angle (angle of diagonal 1-3)
%th_c = atan2(y3 - y1, x3 - x1);

%%
th_c_raw = atan2(y3 - y1, x3 - x1);

if nargin >= 13 && ~isempty(th_c_prev)
    % Unwrap based on previous value
    while (th_c_raw - th_c_prev) > pi
        th_c_raw = th_c_raw - 2*pi;
    end
    while (th_c_raw - th_c_prev) < -pi
        th_c_raw = th_c_raw + 2*pi;
    end
end

th_c = th_c_raw;

%% Remainder of old code
% Angle between diagonals
phi = -atan2(y4 - y2, x4 - x2) + atan2(y3 - y1, x3 - x1);
phi = mod(phi + pi, 2*pi) - pi;

% Intersection ratios using line intersection method
% Solving for where diagonals 1-3 and 2-4 intersect
delta = (x3 - x1) * (y2 - y4) + (y3 - y1) * (x4 - x2);


% Standard intersection calculation
r1 = ((x2 - x1) * (y2 - y4) + (y2 - y1) * (x4 - x2)) / delta;
r2 = ((x3 - x1) * (y2 - y1) - (y3 - y1) * (x2 - x1)) / delta;


% Combining all readings into fwdkin vector
fwdkin = [0 0 0 0 0 0 0 0];
fwdkin(1) = d1;      % Diagonal 1 length
fwdkin(2) = d2;      % Diagonal 2 length  
fwdkin(3) = r1;      % Intersection ratio 1
fwdkin(4) = r2;      % Intersection ratio 2
fwdkin(5) = phi;     % Angle between diagonals
fwdkin(6) = x_c;     % Centroid x
fwdkin(7) = y_c;     % Centroid y
fwdkin(8) = th_c;    % Overall rotation angle

current = [x_c, y_c, d1, d2, th_c, phi, r1, r2];

% Append to existing or create new
persistent FK_results;
persistent call_count;

max_calls = 201; % Set your maximum

% Initialize on first call
if isempty(call_count)
    call_count = 0;
    FK_results = zeros(max_calls, 8);
end

% Increment counter and append data
call_count = call_count + 1;
if call_count <= max_calls
    FK_results(call_count, :) = [x_c, y_c, d1, d2, th_c, phi, r1, r2];
    
    % Save only the filled rows
    assignin('base', 'FK_results', FK_results(1:call_count, :));
end
end
